simulink model "balrob3d_maca64"  (R2019b)
settings: Solver=ode23  StartTime=0.0  StopTime=30  RelTol=1e-3  EnableMultiTasking=on
values from neighbouring files (symbols this model uses):
  g = 9.81    [balrob_params.m]
  x0 = [      0,      5*deg2rad,      0,      0]    [balrob_params.m]
undefined symbols (not defined in the file or in its folder): body, gbox, mot, sens, wheel
Description:
  | Riccardo Antonello (riccardo.antonello@unipd.it)
  | 
  | September 01, 2016
  | 
  | Dept. of Information Engineering, University of Padova
settings Model: Creator=Riccardo  LastModifiedBy=riccardo
settings DataIOCC: LimitDataPoints=on  SaveFormat=Array  ReturnWorkspaceOutputs=off
settings OptimizationCC: LifeSpan=inf
settings DebuggingCC: SolverPrmCheckMsg=warning  SFUnexpectedBacktrackingDiag=warning  SFNoUnconditionalDefaultTransitionDiag=warning  SFExecutionAtInitializationDiag=none  ArithmeticOperatorsInVariantConditions=warning
settings HardwareCC: ProdBitPerPointer=32  ProdBitPerSizeT=32  ProdBitPerPtrDiffT=32  ProdLargestAtomicFloat=None  ProdIntDivRoundTo=Undefined  ProdEndianess=Unspecified  ProdWordSize=32  ProdHWDeviceType=32-bit Generic
settings ModelReferenceCC: PropagateSignalLabelsOutOfModel=off
settings SFSimCC: SimUseLocalCustomCode=off  CustomCodeUndefinedFunction=UseInterfaceOnly
settings RTWCC: RTWUseLocalCustomCode=off
settings CodeAppCC: StateflowObjectComments=on
settings GRTTargetCC: TargetLangStandard=C89/C90 (ANSI)  GeneratePreprocessorConditionals=Disable all
settings ConfigComp: CovMetricSettings=dw  CovHtmlReporting=on  CovSaveCumulativeToWorkspaceVar=on  CovSaveSingleToWorkspaceVar=on  CovExternalEMLEnable=off  CovSFcnEnable=off

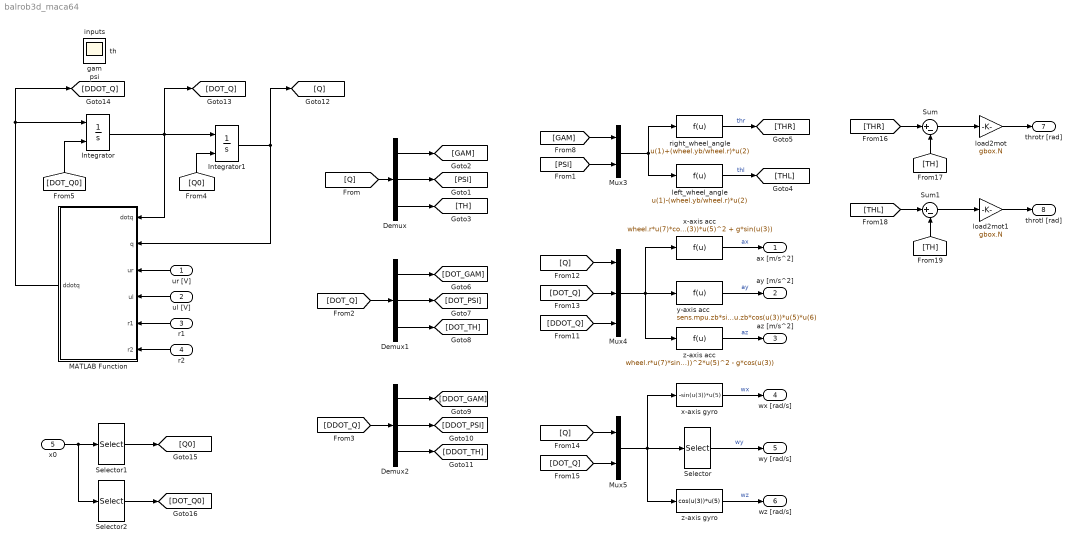
== system balrob3d_maca64 ==
  ur [V] : Inport
  ul [V] : Inport  Port=2
  r1 : Inport  Port=3
  r2 : Inport  Port=4
  x0 : Inport  Port=5
  Demux : Demux  Outputs=3
  Demux1 : Demux  Outputs=3
  Demux2 : Demux  Outputs=3
  Integrator : Integrator  InitialConditionSource=external  InitialCondition=x0(4:6)
  Integrator1 : Integrator  InitialConditionSource=external  InitialCondition=x0(1:3)
  MATLAB Function : MATLAB Function  TreatAsAtomicUnit=on
  Mux3 : Mux  Inputs=2
  Mux4 : Mux  Inputs=3
  Mux5 : Mux  Inputs=2
  Selector : Selector  InputPortWidth=6  IndexOptions=Index vector (dialog)  Indices=6  OutputSizes=1
  Selector1 : Selector  InputPortWidth=6  IndexOptions=Index vector (dialog)  Indices=1:3  OutputSizes=1
  Selector2 : Selector  InputPortWidth=6  IndexOptions=Index vector (dialog)  Indices=4:6  OutputSizes=1
  Sum : Sum  Inputs=|+-
  Sum1 : Sum  Inputs=|+-
  left_wheel_angle : Fcn  Expr=u(1)-(wheel.yb/wheel.r)*u(2)
  load2mot : Gain  Gain=gbox.N
  load2mot1 : Gain  Gain=gbox.N
  right_wheel_angle : Fcn  Expr=u(1)+(wheel.yb/wheel.r)*u(2)
  x-axis acc : Fcn  Expr=wheel.r*u(7)*cos(u(3)) - sens.mpu.yb*cos(u(3))*u(8) + sens.mpu.zb*u(9) - sens.mpu.zb*sin(u(3))*cos(u(3))*u(5)^2 + g*sin(u(3))
  x-axis gyro : Fcn  Expr=-sin(u(3))*u(5)
  y-axis acc : Fcn  Expr=sens.mpu.zb*sin(u(3))*u(7) - sens.mpu.yb*u(5)^2 + wheel.r*u(4)*u(5) + 2*sens.mpu.zb*cos(u(3))*u(5)*u(6)
  z-axis acc : Fcn  Expr=wheel.r*u(7)*sin(u(3)) - sens.mpu.yb*sin(u(3))*u(7) - sens.mpu.zb*u(6)^2 - sens.mpu.zb*sin(u(3))^2*u(5)^2 - g*cos(u(3))
  z-axis gyro : Fcn  Expr=cos(u(3))*u(5)
  ax [m/s^2] : Outport
  ay [m/s^2] : Outport  Port=2
  az [m/s^2] : Outport  Port=3
  wx [rad/s] : Outport  Port=4
  wy [rad/s] : Outport  Port=5
  wz [rad/s] : Outport  Port=6
  throtr [rad] : Outport  Port=7
  throtl [rad] : Outport  Port=8
  gam : Scope
  inputs : Scope
  psi : Scope
  th : Scope
  wires:
  left_wheel_angle/1 -> [THL]  "thl"
  Mux3/1 -> left_wheel_angle/1, right_wheel_angle/1
  right_wheel_angle/1 -> [THR]  "thr"
  [GAM] -> Mux3/1
  [PSI] -> Mux3/2
  [DOT_Q] -> Mux4/2
  [DDOT_Q] -> Mux4/3
  [Q] -> Mux4/1
  z-axis gyro/1 -> wz [rad/s]/1  "wz"
  x-axis gyro/1 -> wx [rad/s]/1  "wx"
  Mux4/1 -> z-axis acc/1, x-axis acc/1, y-axis acc/1
  x-axis acc/1 -> ax [m/s^2]/1  "ax"
  y-axis acc/1 -> ay [m/s^2]/1  "ay"
  z-axis acc/1 -> az [m/s^2]/1  "az"
  [Q] -> Mux5/1
  [DOT_Q] -> Mux5/2
  Mux5/1 -> z-axis gyro/1, x-axis gyro/1, Selector/1
  Selector/1 -> wy [rad/s]/1  "wy"
  [THR] -> Sum/1
  [TH] -> Sum/2
  Sum/1 -> load2mot/1
  Sum1/1 -> load2mot1/1
  [TH] -> Sum1/2
  [THL] -> Sum1/1
  load2mot1/1 -> throtl [rad]/1
  ur [V]/1 -> MATLAB Function/3(ur)
  ul [V]/1 -> MATLAB Function/4(ul)
  Demux/2 -> [PSI]
  Demux/1 -> [GAM]
  Demux/3 -> [TH]
  Demux1/1 -> [DOT_GAM]
  Demux1/2 -> [DOT_PSI]
  Demux1/3 -> [DOT_TH]
  Demux2/1 -> [DDOT_GAM]
  Demux2/2 -> [DDOT_PSI]
  Demux2/3 -> [DDOT_TH]
  [Q] -> Demux/1
  [DOT_Q] -> Demux1/1
  [DDOT_Q] -> Demux2/1
  Integrator1/1 -> [Q], MATLAB Function/2(q)
  Integrator/1 -> MATLAB Function/1(dotq), [DOT_Q], Integrator1/1
  MATLAB Function/1(ddotq) -> [DDOT_Q], Integrator/1
  load2mot/1 -> throtr [rad]/1
  r1/1 -> MATLAB Function/5(r1)
  r2/1 -> MATLAB Function/6(r2)
  x0/1 -> Selector2/1, Selector1/1
  Selector1/1 -> [Q0]
  Selector2/1 -> [DOT_Q0]
  [Q0] -> Integrator1/2
  [DOT_Q0] -> Integrator/2

== matlab function balrob3d_maca64/MATLAB Function ==
  data: dotq input; q input; ur input; ddotq output size=3; ul input; r1 input; r2 input; body parameter; mot parameter; gbox parameter; wheel parameter
function ddotq = fcn(dotq, q, ur, ul, r1, r2, body, mot, gbox, wheel)

%%  Extract state components

th = q(3);

dot_gam = dotq(1);
dot_psi = dotq(2);
dot_th  = dotq(3);


%%  Extract params

%   body params
l       = body.zb;
mb      = body.m;
Ibxx    = body.Ixx;
Ibyy    = body.Iyy;
Ibzz    = body.Izz;

%   wheel params
w       = 2*wheel.yb;
r       = wheel.r;
mw      = wheel.m;
% Iwxx    = wheel.Ixx;
Iwyy    = wheel.Iyy;
Iwzz    = wheel.Izz;

%   (motor) rotor params
ybrot   = mot.rot.yb; 
zbrot   = mot.rot.zb;
mrot    = mot.rot.m;
Irotxx  = mot.rot.Ixx;
Irotyy  = mot.rot.Iyy;
Irotzz  = mot.rot.Izz;

%   gear ratio
n   = gbox.N;

%   friction params
bw  = wheel.B;      %   wheel viscous fric coeff
bm  = mot.B;        %   motor viscous fric coeff (motor side)
bg  = gbox.B;       %   gbox viscous fric coeff (load side)
b   = n^2*bm+bg;    %   motor+gbox viscous fric coeff (load side)

%   gravity acc
g = 9.81;


%%  Get motor torques

%   wheel speeds
dot_thr = dot_gam + (w/2/r)*dot_psi;
dot_thl = dot_gam - (w/2/r)*dot_psi;

%   back-EMFs
uer = mot.Ke * n*(dot_thr-dot_th);
uel = mot.Ke * n*(dot_thl-dot_th);

%   motor currents
iar = (ur-uer)/mot.R;
ial = (ul-uel)/mot.R;

%   motor torques
taur = n*mot.Kt * iar;
taul = n*mot.Kt * ial;


%%  Get friction torques

%   nominal friction torque
taufr = gbox.B*(dot_thr-dot_th) + gbox.tausf*sign(dot_thr-dot_th);
taufl = gbox.B*(dot_thl-dot_th) + gbox.tausf*sign(dot_thl-dot_th);

%   add random deviation from nominal value
taufr = r1*taufr;
taufl = r2*taufl;


%%  Overall torques

taur = taur - taufr;
taul = taul - taufl;


%%  Evaluate accelerations of generalised coords

%   inertia matrix 
BB = zeros(3,3);
BB(1,1) = 2*Iwyy + 2*Irotyy*n^2+(mb + 2*(mrot+mw))*r^2;
BB(1,2) = 0;
BB(1,3) = 2*(1-n)*n*Irotyy + r*(l*mb + 2*mrot*zbrot)*cos(th);

BB(2,1) = 0;
BB(2,2) = 2*(Iwyy + Irotyy*n^2)*(w/2/r)^2 + ...
	(1/2)*(Ibxx + Ibzz + 2*Irotxx + 2*Irotzz + 4*Iwzz + mb*l^2 + mw*w^2 + 4*mrot*ybrot^2 + 2*mrot*zbrot^2) - ...
	(1/2)*(Ibxx - Ibzz + 2*Irotxx - 2*Irotzz + mb*l^2 + 2*mrot*zbrot^2)*cos(th);
BB(2,3) = 0;

BB(3,1) = BB(1,3);
BB(3,2) = 0;
BB(3,3) = Ibyy + mb*l^2 + 2*(1-n)^2*Irotyy + 2*mrot*zbrot^2;


%   Coriolis + centrifugal terms matrix
CC = zeros(3,3);
CC(1,1) = 0;
CC(1,2) = 0;
CC(1,3) = -r*(mb*l + 2*mrot*zbrot)*sin(th)*dot_th;

aux = (1/2)*(Ibxx - Ibzz + 2*Irotxx - 2*Irotzz + mb*l^2 + 2*mrot*zbrot^2)*sin(2*th);
CC(2,1) = 0;
CC(2,2) = aux*dot_th;
CC(2,3) = aux*dot_psi;

CC(3,1) = 0;
CC(3,2) = -CC(2,3);
CC(3,3) = 0;


%   viscous friction matrix
Fv = zeros(3,3);
% Fv(1,1) = 2*(b+bw);
% Fv(1,2) = 0;
% Fv(1,3) = -2*b;
% 
% Fv(2,1) = 0;
% Fv(2,2) = 2*(b+bw)*(w/2/r)^2;
% Fv(2,3) = 0;
% 
% Fv(3,1) = -2*b;
% Fv(3,2) = 0;
% Fv(3,3) = 2*b;


%   gravity loading
GG = zeros(3,1);
GG(3) = -g*(mb*l + 2*mrot*zbrot)*sin(th);


%   generalized actuator forces
HH = zeros(3,1);
HH(1) = taur + taul;
HH(2) = (w/2/r)*(taur - taul);
HH(3) = -(taur + taul);


%   get accelerations of generalised coords
% q = [gam, psi, th].';
dotq = [dot_gam, dot_psi, dot_th].';
ddotq = BB \ (HH - CC*dotq - Fv*dotq - GG);
